simulink model "simu2022a"  (R2022a)
settings: Solver=ode1  StartTime=0.0  StopTime=Tstop  FixedStep=dt  RelTol=1e-3
values from neighbouring files (symbols this model uses):
  N = dim2 / 2    [animation1.m]    (also in cbf_centralized.m = 10; cbf_decentralized.m = 7; centralized_cbf_step.m = evalin('base', 'N'); hybrid_cbf_step.m = evalin('base','N'))
settings Model: Creator=Filippo  LastModifiedBy=Filippo
settings DataIOCC: ReturnWorkspaceOutputs=off
settings ModelReferenceCC: EnableRefExpFcnMdlSchedulingChecks=off
settings RTWCC: Description=Generic Real-Time Target  GPUComputeCapability=5.0
settings ConfigComp: CovBoundaryAbsTol=1.0e-5

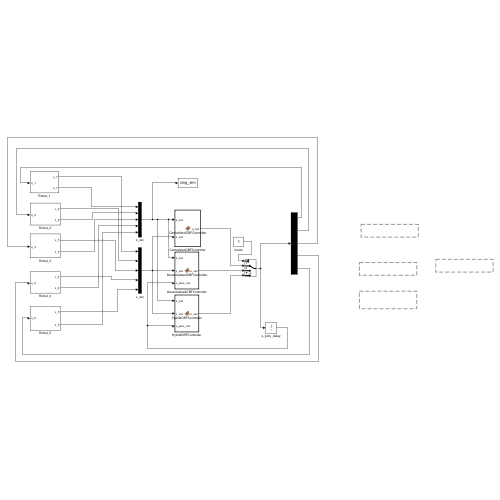
[thumbnail: Simulink's stored preview of the top-level diagram]
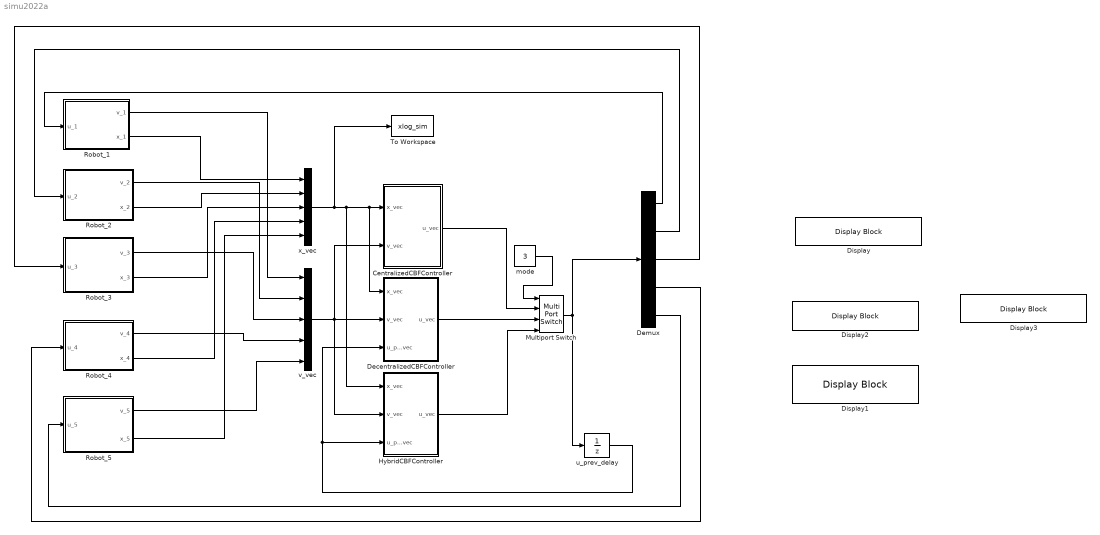
== system simu2022a ==
  CentralizedCBFController : MATLAB Function  TreatAsAtomicUnit=on
  DecentralizedCBFController : MATLAB Function  TreatAsAtomicUnit=on
  Demux : Demux  Outputs=5
  Display{,1..3} (4 alike) : DisplayBlock  LabelPosition=Hide  Transparency=1
  HybridCBFController : MATLAB Function  TreatAsAtomicUnit=on
  Multiport Switch : MultiPortSwitch  SaturateOnIntegerOverflow=off  InputSameDT=off
  Robot_1 : Subsystem
  Robot_2 : Subsystem
  Robot_3 : Subsystem
  Robot_4 : Subsystem
  Robot_5 : Subsystem
  To Workspace : ToWorkspace  VariableName=xlog_sim  SampleTime=-1
  mode : Constant  Value=3
  u_prev_delay : UnitDelay  InitialCondition=zeros(2*N,1)  SampleTime=-1  HasFrameUpgradeWarning=on
  v_vec : Mux  Inputs=5
  x_vec : Mux  Inputs=5
  wires:
  CentralizedCBFController/1(u_vec) -> Multiport Switch/2
  u_prev_delay/1 -> HybridCBFController/3(u_prev_vec), DecentralizedCBFController/3(u_prev_vec)
  mode/1 -> Multiport Switch/1
  HybridCBFController/1(u_vec) -> Multiport Switch/4
  Multiport Switch/1 -> Demux/1, u_prev_delay/1
  DecentralizedCBFController/1(u_vec) -> Multiport Switch/3
  Robot_1/2(x_1) -> x_vec/1
  Robot_2/2(x_2) -> x_vec/2
  Robot_3/2(x_3) -> x_vec/3
  Robot_4/2(x_4) -> x_vec/4
  Robot_5/2(x_5) -> x_vec/5
  Robot_1/1(v_1) -> v_vec/1
  Robot_2/1(v_2) -> v_vec/2
  Robot_3/1(v_3) -> v_vec/3
  Robot_4/1(v_4) -> v_vec/4
  Robot_5/1(v_5) -> v_vec/5
  x_vec/1 -> To Workspace/1, HybridCBFController/1(x_vec), DecentralizedCBFController/1(x_vec), CentralizedCBFController/1(x_vec)
  v_vec/1 -> CentralizedCBFController/2(v_vec), HybridCBFController/2(v_vec), DecentralizedCBFController/2(v_vec)
  Demux/5 -> Robot_5/1(u_5)
  Demux/1 -> Robot_1/1(u_1)
  Demux/4 -> Robot_4/1(u_4)
  Demux/3 -> Robot_3/1(u_3)
  Demux/2 -> Robot_2/1(u_2)

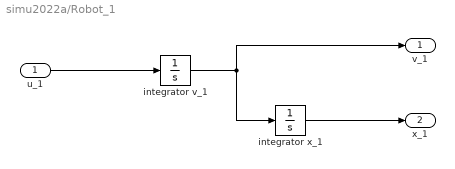
== system simu2022a/Robot_1 ==
  u_1 : Inport
  integrator v_1 : Integrator  InitialCondition=[0; 0]
  integrator x_1 : Integrator  InitialCondition=|
      | [ 6.0;
      |   0.0 ]
  v_1 : Outport
  x_1 : Outport  Port=2
  wires:
  integrator v_1/1 -> v_1/1, integrator x_1/1
  u_1/1 -> integrator v_1/1
  integrator x_1/1 -> x_1/1

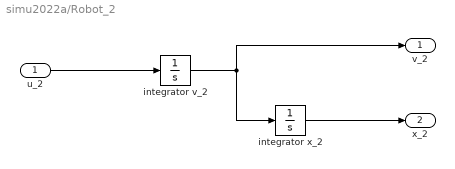
== system simu2022a/Robot_2 ==
  u_2 : Inport
  integrator v_2 : Integrator  InitialCondition=[0; 0]
  integrator x_2 : Integrator  InitialCondition=|
      | [ 1.85;
      |   5.71 ]
  v_2 : Outport
  x_2 : Outport  Port=2
  wires:
  integrator v_2/1 -> v_2/1, integrator x_2/1
  u_2/1 -> integrator v_2/1
  integrator x_2/1 -> x_2/1

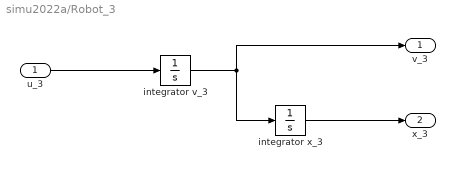
== system simu2022a/Robot_3 ==
  u_3 : Inport
  integrator v_3 : Integrator  InitialCondition=[0; 0]
  integrator x_3 : Integrator  InitialCondition=|
      | [ -4.85;
      |    3.53 ]
  v_3 : Outport
  x_3 : Outport  Port=2
  wires:
  integrator v_3/1 -> v_3/1, integrator x_3/1
  u_3/1 -> integrator v_3/1
  integrator x_3/1 -> x_3/1

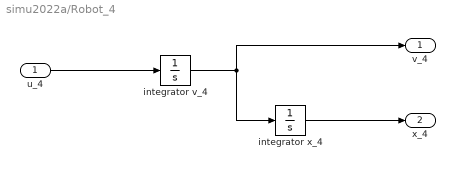
== system simu2022a/Robot_4 ==
  u_4 : Inport
  integrator v_4 : Integrator  InitialCondition=[0; 0]
  integrator x_4 : Integrator  InitialCondition=|
      | [ -4.85;
      |   -3.53 ]
  v_4 : Outport
  x_4 : Outport  Port=2
  wires:
  integrator v_4/1 -> v_4/1, integrator x_4/1
  u_4/1 -> integrator v_4/1
  integrator x_4/1 -> x_4/1

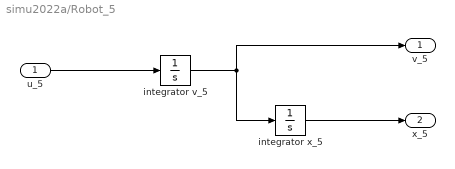
== system simu2022a/Robot_5 ==
  u_5 : Inport
  integrator v_5 : Integrator  InitialCondition=[0; 0]
  integrator x_5 : Integrator  InitialCondition=|
      | [ 1.85;
      |  -5.71 ]
  v_5 : Outport
  x_5 : Outport  Port=2
  wires:
  integrator v_5/1 -> v_5/1, integrator x_5/1
  u_5/1 -> integrator v_5/1
  integrator x_5/1 -> x_5/1

== matlab function simu2022a/CentralizedCBFController ==
  data: x_vec input; u_vec output; v_vec input
function u_vec = CentralizedCBFController(x_vec, v_vec)
%#codegen
% Wrapper per chiamare la funzione esterna centralized_cbf_step
% dallo schema Simulink.

    coder.extrinsic('centralized_cbf_step');   % dico al coder che è una funzione MATLAB "normale"

    % Per permettere a Simulink di capire le dimensioni, prealloca u_vec
    % N = 5 --> 2N = 10. Se vuoi usare N dal workspace:
    %   coder.extrinsic('evalin');
    %   N = evalin('base','N');
    %   u_vec = zeros(2*N,1);
    N = 5;              % <-- se ora stai lavorando con 5 robot
    u_vec = zeros(2*N,1);

    % Chiamata vera e propria alla funzione di controllo
    u_vec = centralized_cbf_step(x_vec, v_vec);
end

== matlab function simu2022a/HybridCBFController ==
  data: x_vec input; u_vec output; v_vec input; u_prev_vec input
function u_vec = HybridCBFController(x_vec, v_vec, u_prev_vec)
%#codegen
% Wrapper per hybrid_cbf_step.m

coder.extrinsic('hybrid_cbf_step');

% per inferenza dimensioni
N = 5;              % oppure leggi dal base workspace con evalin se vuoi
u_vec = zeros(2*N,1);

u_vec = hybrid_cbf_step(x_vec, v_vec, u_prev_vec);
end

== matlab function simu2022a/DecentralizedCBFController ==
  data: x_vec input; u_vec output; v_vec input; u_prev_vec input
function u_vec = DecentralizedCBFController(x_vec, v_vec, u_prev_vec)
%#codegen
% Wrapper per chiamare decentralized_cbf_step da Simulink

coder.extrinsic('decentralized_cbf_step');

% Numero agenti (qui puoi fissare N=5 o leggere dal base workspace)
N = 5;                     % oppure usa evalin se vuoi:
% coder.extrinsic('evalin');
% N = evalin('base','N');

u_vec = zeros(2*N,1);      % per inferenza dimensioni

u_vec = decentralized_cbf_step(x_vec, v_vec, u_prev_vec);
end
